simulink model "model"  (R2022a)
settings: Solver=FixedStepDiscrete  StartTime=0.0  StopTime=Inf  FixedStep=5e-3  RelTol=1e-3
values from neighbouring files (symbols this model uses):
  emin = 0.05    [simulate.m]
  gamma = 0.3    [simulate.m]
  k = 1    [simulate.m]
  omega_max = (pi/180)*300    (= 5.23598775598)    [simulate.m]
  u_max = 1.2    [simulate.m]
libraries: fuzblock x3, simulink x1
settings Model: Creator=mateu  LastModifiedBy=mateu
settings SFSimCC: SimTargetLang=C++

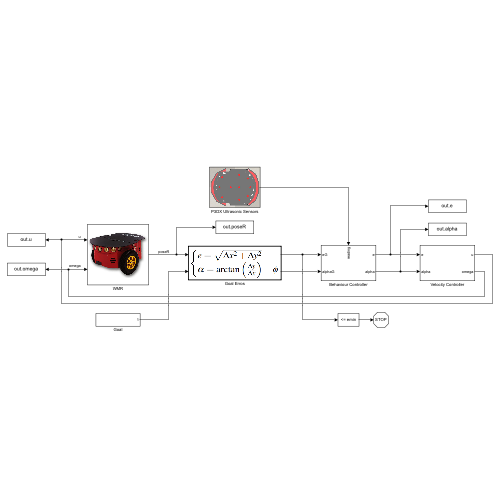
[thumbnail: Simulink's stored preview of the top-level diagram]
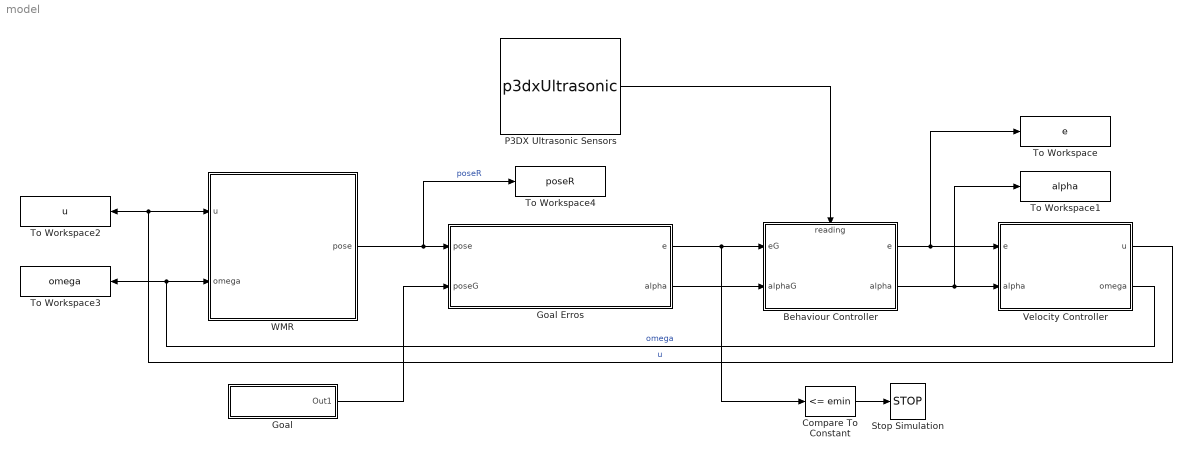
== system model ==
  Behaviour Controller : Subsystem
      settings: PortSchema="{\"entries\":[{\"content\":{\"sides\":[{\"content\":{\"connectorIds\":[\"In1\",\"In2\"]},\"type\":\"ConnectorPlacement.EquallySpacedRectSide\",\"uuid\":\"06a7f3f5-19ad-4266-b822-3ab888d38f4d\"},{\"content\":{\"connectorIds\":[\"Out1\",\"Out2\"],\"side\":\"RIGHT\"},\"type\":\"ConnectorPlacement.EquallySpacedRectSide\",\"uuid\":\"a9a64b0c-d306-4cfa-a00f-170269f42e3e\"},{\"content\":{\"connectorIds\":[\"In3\"],\"side\":\"TOP\"},\"type\":\"ConnectorPlacement.EquallySpacedRectSide\",\"uuid\":\"e45decad-4705-465d-8cfa-5faf0b21f90f\"}]},\"type\":\"ConnectorPlacement.EquallySpacedConnector\",\"uuid\":\"b00d1ded-7e91-4878-9283-b58fef4283ca\"}],\"packageUris\":[\"http://schema.mathworks.com/mf0/Connector/R2020b\"],\"version\":\"1.0\"}"
  Compare To Constant : simulink/Logic and Bit Operations/Compare To Constant  relop=<=  const=emin  OutDataTypeStr=boolean
  Goal : Subsystem  VariantControl=GOAL_COPPELIA
  Goal Erros : MATLAB Function  TreatAsAtomicUnit=on
  P3DX Ultrasonic Sensors : M-S-Function  FunctionName=p3dxUltrasonic
      mask Display: image('$imagefile'); % Use "Edit Image" on toolstrip to change.
  Stop Simulation : Stop
  To Workspace : ToWorkspace  VariableName=e  SaveFormat=Timeseries  SampleTime=-1
  To Workspace1 : ToWorkspace  VariableName=alpha  SaveFormat=Timeseries  SampleTime=-1
  To Workspace2 : ToWorkspace  VariableName=u  SaveFormat=Timeseries  SampleTime=-1
  To Workspace3 : ToWorkspace  VariableName=omega  SaveFormat=Timeseries  SampleTime=-1
  To Workspace4 : ToWorkspace  VariableName=poseR  SaveFormat=Timeseries  SampleTime=-1
  Velocity Controller : Subsystem
  WMR : Subsystem  VariantControl=UNICYCLE_COPPELIA
      mask Display: image('$imagefile'); % Use "Edit Image" on toolstrip to change.
  wires:
  WMR/1(pose) -> To Workspace4/1, Goal Erros/1(pose)  "poseR"
  Goal/1(Out1) -> Goal Erros/2(poseG)
  Compare To Constant/1 -> Stop Simulation/1
  Velocity Controller/1(u) -> WMR/1(u), To Workspace2/1  "u"
  Velocity Controller/2(omega) -> WMR/2(omega), To Workspace3/1  "omega"
  Goal Erros/1(e) -> Behaviour Controller/1(eG), Compare To Constant/1
  Goal Erros/2(alpha) -> Behaviour Controller/2(alphaG)
  P3DX Ultrasonic Sensors/1 -> Behaviour Controller/3(reading)
  Behaviour Controller/1(e) -> Velocity Controller/1(e), To Workspace/1
  Behaviour Controller/2(alpha) -> Velocity Controller/2(alpha), To Workspace1/1

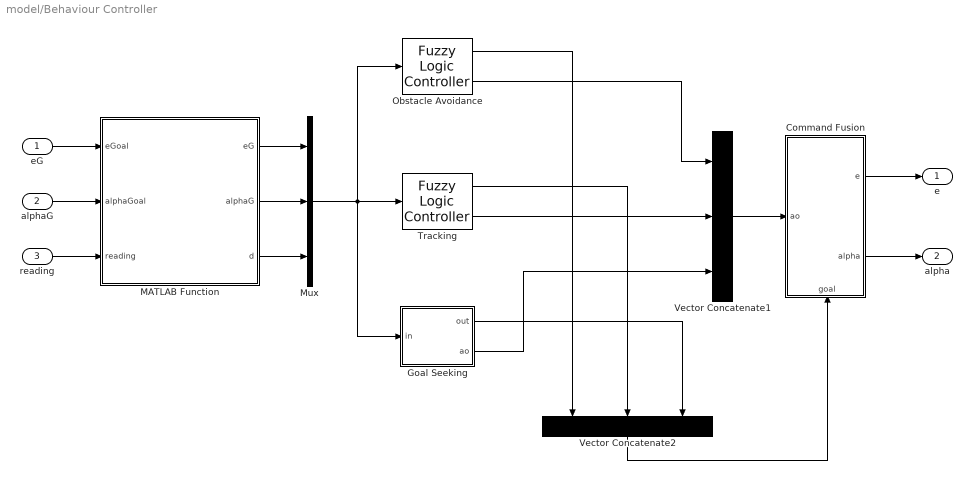
== system model/Behaviour Controller ==
  eG : Inport
  alphaG : Inport  Port=2
  reading : Inport  Port=3
  Command Fusion : Subsystem
      settings: PortSchema="{\"entries\":[{\"content\":{\"sides\":[{\"content\":{\"connectorIds\":[\"In1\"]},\"type\":\"ConnectorPlacement.EquallySpacedRectSide\",\"uuid\":\"73fd97c8-3045-4cbb-bad3-62703d9c5625\"},{\"content\":{\"connectorIds\":[\"Out1\",\"Out2\"],\"side\":\"RIGHT\"},\"type\":\"ConnectorPlacement.EquallySpacedRectSide\",\"uuid\":\"597553a6-e8ee-4dcc-95be-8e7ec85d134a\"},{\"content\":{\"connectorIds\":[],\"side\":\"TOP\"},\"type\":\"ConnectorPlacement.EquallySpacedRectSide\",\"uuid\":\"405b4f83-372d-4f6d-b03d-1931eb808694\"},{\"content\":{\"connectorIds\":[\"In2\"],\"side\":\"BOTTOM\"},\"type\":\"ConnectorPlacement.EquallySpacedRectSide\",\"uuid\":\"64f45c17-9083-4d96-bfee-fa5f6d303fa3\"}]},\"type\":\"ConnectorPlacement.EquallySpacedConnector\",\"uuid\":\"7fff97a2-a0c4-49e1-9e26-ea35b77b3e7f\"}],\"packageUris\":[\"http://schema.mathworks.com/mf0/Connector/R2020b\"],\"version\":\"1.0\"}"
  Goal Seeking : Subsystem
  MATLAB Function : MATLAB Function  TreatAsAtomicUnit=on
  Mux : Mux  Inputs=3
  Obstacle Avoidance : fuzblock/Fuzzy Logic  Controller  FIS=fisOA  OutputSampleNumber=101  DataType=double  FuzzifiedInputs=off  RuleFiringStrengths=off  RuleOutputs=off  AggregatedOutputs=on  SimulateUsing=Interpreted execution  OutOfRangeInputValueMessage=none  NoRuleFiredMessage=none  EmptyOutputFuzzySetMessage=none
  Tracking : fuzblock/Fuzzy Logic  Controller  FIS=fisTR  OutputSampleNumber=101  DataType=double  FuzzifiedInputs=off  RuleFiringStrengths=off  RuleOutputs=off  AggregatedOutputs=on  SimulateUsing=Interpreted execution  OutOfRangeInputValueMessage=none  NoRuleFiredMessage=none  EmptyOutputFuzzySetMessage=none
  Vector Concatenate1 : Concatenate  NumInputs=3  Mode=Multidimensional array  ConcatenateDimension=2
  Vector Concatenate2 : Concatenate  NumInputs=3  Mode=Multidimensional array  ConcatenateDimension=2
  e : Outport
  alpha : Outport  Port=2
  wires:
  Mux/1 -> Goal Seeking/1(in), Obstacle Avoidance/1, Tracking/1
  reading/1 -> MATLAB Function/3(reading)
  MATLAB Function/2(alphaG) -> Mux/2
  MATLAB Function/1(eG) -> Mux/1
  alphaG/1 -> MATLAB Function/2(alphaGoal)
  eG/1 -> MATLAB Function/1(eGoal)
  MATLAB Function/3(d) -> Mux/3
  Command Fusion/1(e) -> e/1
  Command Fusion/2(alpha) -> alpha/1
  Obstacle Avoidance/2 -> Vector Concatenate1/1
  Tracking/2 -> Vector Concatenate1/2
  Vector Concatenate1/1 -> Command Fusion/1(ao)
  Obstacle Avoidance/1 -> Vector Concatenate2/1
  Tracking/1 -> Vector Concatenate2/2
  Goal Seeking/1(out) -> Vector Concatenate2/3
  Vector Concatenate2/1 -> Command Fusion/2(goal)
  Goal Seeking/2(ao) -> Vector Concatenate1/3

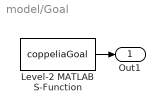
== system model/Goal ==
  Level-2 MATLAB S-Function : M-S-Function  FunctionName=coppeliaGoal
  Out1 : Outport
  wires:
  Level-2 MATLAB S-Function/1 -> Out1/1

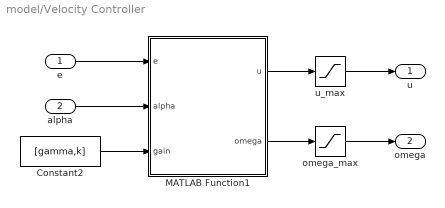
== system model/Velocity Controller ==
  e : Inport
  alpha : Inport  Port=2
  Constant2 : Constant  Value=[gamma,k]
  MATLAB Function1 : MATLAB Function  TreatAsAtomicUnit=on
  omega_max : Saturate  UpperLimit=omega_max  LowerLimit=-omega_max
  u_max : Saturate  UpperLimit=u_max  LowerLimit=-u_max
  u : Outport
  omega : Outport  Port=2
  wires:
  Constant2/1 -> MATLAB Function1/3(gain)
  omega_max/1 -> omega/1
  u_max/1 -> u/1
  alpha/1 -> MATLAB Function1/2(alpha)
  e/1 -> MATLAB Function1/1(e)
  MATLAB Function1/2(omega) -> omega_max/1
  MATLAB Function1/1(u) -> u_max/1

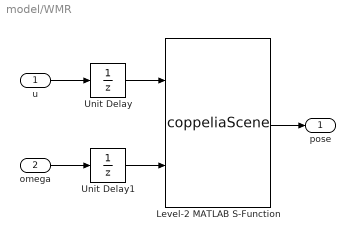
== system model/WMR ==
  u : Inport
  omega : Inport  Port=2
  Level-2 MATLAB S-Function : M-S-Function  FunctionName=coppeliaScene
  Unit Delay : UnitDelay  SampleTime=-1  HasFrameUpgradeWarning=on
  Unit Delay1 : UnitDelay  SampleTime=-1  HasFrameUpgradeWarning=on
  pose : Outport
  wires:
  u/1 -> Unit Delay/1
  omega/1 -> Unit Delay1/1
  Level-2 MATLAB S-Function/1 -> pose/1
  Unit Delay/1 -> Level-2 MATLAB S-Function/1
  Unit Delay1/1 -> Level-2 MATLAB S-Function/2

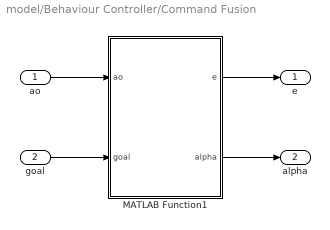
== system model/Behaviour Controller/Command Fusion ==
  ao : Inport
  goal : Inport  Port=2
  MATLAB Function1 : MATLAB Function  TreatAsAtomicUnit=on
  e : Outport
  alpha : Outport  Port=2
  wires:
  ao/1 -> MATLAB Function1/1(ao)
  MATLAB Function1/2(alpha) -> alpha/1
  MATLAB Function1/1(e) -> e/1
  goal/1 -> MATLAB Function1/2(goal)

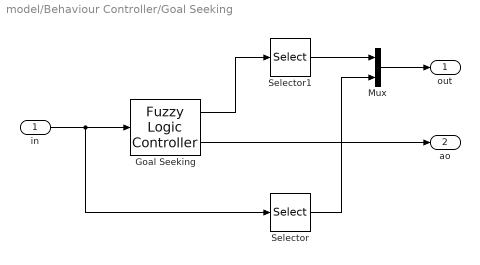
== system model/Behaviour Controller/Goal Seeking ==
  in : Inport
  Goal Seeking : fuzblock/Fuzzy Logic  Controller  FIS=fisGS  OutputSampleNumber=101  DataType=double  FuzzifiedInputs=off  RuleFiringStrengths=off  RuleOutputs=off  AggregatedOutputs=on  SimulateUsing=Interpreted execution  OutOfRangeInputValueMessage=none  NoRuleFiredMessage=none  EmptyOutputFuzzySetMessage=none
  Mux : Mux  Inputs=2
  Selector : Selector  InputPortWidth=5  IndexOptions=Index vector (dialog)  Indices=[2]  OutputSizes=1
  Selector1 : Selector  InputPortWidth=2  IndexOptions=Index vector (dialog)  Indices=[1]  OutputSizes=1
  out : Outport
  ao : Outport  Port=2
  wires:
  in/1 -> Goal Seeking/1, Selector/1
  Goal Seeking/1 -> Selector1/1
  Selector/1 -> Mux/2
  Selector1/1 -> Mux/1
  Mux/1 -> out/1
  Goal Seeking/2 -> ao/1

== matlab function model/Behaviour Controller/MATLAB Function ==
  data: eGoal input; alphaGoal input; eG output; alphaG output; reading input size=16; d output
function [eG,alphaG,d] = inputGen(eGoal,alphaGoal,reading)

idx = [[3 4 5 6];[7 8 9 7];[2 1 16 2]];

d = zeros(1,3); r = zeros(1,4);
for i = 1:3
    r = reading(idx(i,:))/2;
    d(i) = min(r);
end
eG = min(eGoal,3);
alphaG = alphaGoal;

== matlab function model/Goal Erros ==
  settings: updateMethod=DISCRETE  sampleTime=0.05
  data: pose input; e output; poseG input; alpha output
function [e,alpha] = errors(pose,poseG)

deltaX = poseG(1)-pose(1); deltaY = poseG(2)-pose(2);
phi = pose(3);

e = sqrt(deltaX^2 + deltaY^2);
alpha = atan2(deltaY,deltaX) - phi;

if alpha < -pi
    alpha = alpha + 2*pi;
elseif alpha >= pi
    alpha = alpha - 2*pi;
end

== matlab function model/Velocity Controller/MATLAB Function1 ==
  settings: updateMethod=DISCRETE  sampleTime=0.05
  data: e input; u output; alpha input; omega output; gain input
function [u,omega] = control(e,alpha,gain)

gamma = gain(1); k = gain(2);

u = gamma*e*cos(alpha);
omega = k*alpha + gamma*cos(alpha)*sin(alpha);

== matlab function model/Behaviour Controller/Command Fusion/MATLAB Function1 ==
  data: ao input; e output; alpha output; goal input
function [e,alpha] = commandFusion(ao,goal)

coder.extrinsic('plotV');
coder.extrinsic('paretto');

w = paretto(max(ao(:,1:2:(end-1)),ao(:,2:2:end)))

e = 0; alpha = 0;
e       = goal(1,:)*w'/sum(w);
alpha   = goal(2,:)*w'/sum(w);

plotV([[e;alpha],goal]);
